simulink model "BLDCctrlBasedOnMBDPILmodel"  (R2020b)
settings: Solver=FixedStepDiscrete  StartTime=0.0  StopTime=10.0  FixedStep=0.0001  RelTol=1e-3
InitFcn:
  | mbd_s32k_consistency_checks(bdroot(gcs));
undefined symbols (not defined in the file or in its folder): LQFP
libraries: mbd_s32k1xx_ec_toolbox x16
settings Model: Creator=k  LastModifiedBy=k
settings DataIOCC: ExternalInput=off  InitialState=off  SaveOutput=off  SignalLogging=off  SaveTime=off
settings OptimizationCC: DefaultParameterBehavior=Inlined  EnhancedBackFolding=on  PassReuseOutputArgsAs=Individual arguments  ZeroExternalMemoryAtStartup=off  ZeroInternalMemoryAtStartup=off  OptimizeBlockOrder=speed  DifferentSizesBufferReuse=on  OptimizationCustomize=off  EfficientTunableParamExpr=on
settings DebuggingCC: InheritedTsInSrcMsg=none  SingleTaskRateTransMsg=error  ParameterTunabilityLossMsg=error  UnconnectedInputMsg=error  UnconnectedOutputMsg=error  UnconnectedLineMsg=error  UnknownTsInhSupMsg=error
settings HardwareCC: ProdBitPerPointer=32  ProdBitPerSizeT=32  ProdBitPerPtrDiffT=32  ProdLargestAtomicInteger=Long  ProdLargestAtomicFloat=Double  ProdWordSize=32  ProdHWDeviceType=ARM Compatible->ARM Cortex
settings SFSimCC: MATLABDynamicMemAlloc=off
settings RTWCC: Description=Model Based Design Toolbox S32K1xx Code Generation Target  SystemTargetFile=mbd_s32k.tlc  MakeCommand=mbd_s32k_make_rtw COPY_MDLREF_INCLUDES=0  TemplateMakefile=mbd_s32k.tmf
settings CodeAppCC: ForceParamTrailComments=on  IgnoreCustomStorageClasses=off  OperatorAnnotations=on  SimulinkDataObjDesc=on  SFDataObjDesc=on  InsertBlockDesc=on
settings STFCustomTargetCC: TargetLangStandard=C99 (ISO)  MultiwordLength=256  ConcurrentExecutionCompliant=off  CombineOutputUpdateFcns=on  ERTCustomFileBanners=on  SupportContinuousTime=off  SupportNonInlinedSFcns=off  RemoveResetFunc=on  MATLABClassNameForMDSCustomization=Simulink.SoftwareTarget.ERTCustomization  CPPClassGenCompliant=off  GRTInterface=off  SystemTargetFile=mbd_s32k.tlc
settings ERTTargetCC: TargetLangStandard=C99 (ISO)  ParMdlRefBuildCompliant=off  CompOptLevelCompliant=off  ConcurrentExecutionCompliant=off  ModelStepFunctionPrototypeControlCompliant=off  CPPClassGenCompliant=off  UseToolchainInfoCompliant=off  InlinedParameterPlacement=NonHierarchical  ERTSrcFileBannerTemplate=mbd_ert_code_template.cgt  ERTHdrFileBannerTemplate=mbd_ert_code_template.cgt  ERTDataSrcFileTemplate=mbd_ert_code_template.cgt  ERTDataHdrFileTemplate=mbd_ert_code_template.cgt  ERTCustomFileTemplate=example_file_process.tlc

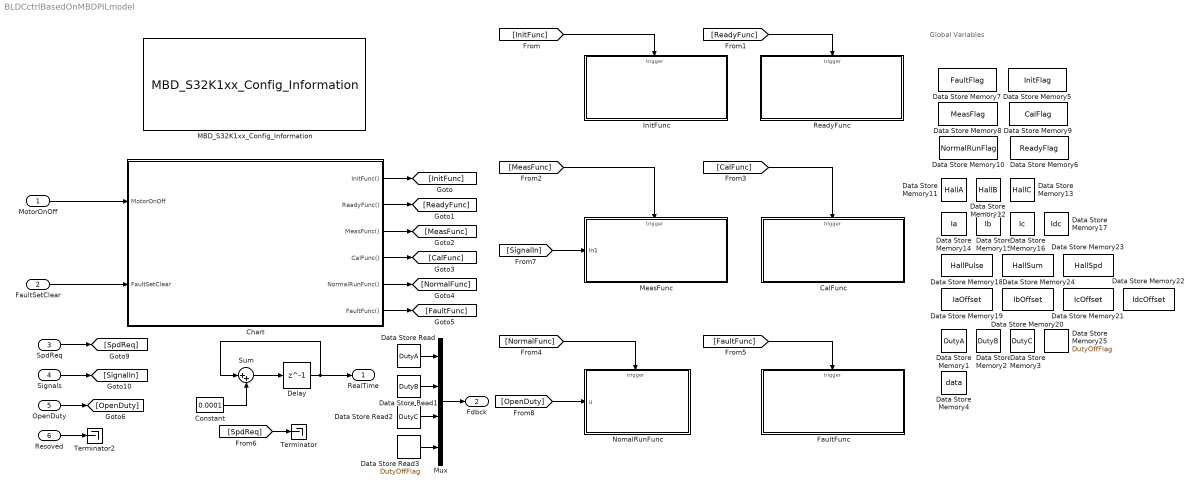
== system BLDCctrlBasedOnMBDPILmodel ==
  note: Global Variables
  MotorOnOff : Inport  OutDataTypeStr=boolean
  FaultSetClear : Inport  Port=2  OutDataTypeStr=boolean
  SpdReq : Inport  Port=3  OutDataTypeStr=single
  Signals : Inport  Port=4  OutDataTypeStr=single  PortDimensions=7
  OpenDuty : Inport  Port=5  OutDataTypeStr=single
  Resoved : Inport  Port=6  OutDataTypeStr=single
  CalFunc : Subsystem  TreatAsAtomicUnit=on
  Chart : Stateflow chart  TreatAsAtomicUnit=on
      settings: PortSchema="{\"entries\":[{\"content\":{\"sides\":[{\"content\":{\"connectorIds\":[\"In1\",\"In2\"]},\"type\":\"ConnectorPlacement.EquallySpacedRectSide\",\"uuid\":\"6aab3670-dbd5-4778-9051-de706f320d6c\"},{\"content\":{\"connectorIds\":[\"Out2\",\"Out3\",\"Out1\",\"Out4\",\"Out5\",\"Out6\"],\"side\":\"RIGHT\"},\"type\":\"ConnectorPlacement.EquallySpacedRectSide\",\"uuid\":\"2f9f0170-7a01-4f36-b182-da63b20b6c86\"},{\"content\":{\"connectorIds\":[],\"side\":\"TOP\"},\"type\":\"ConnectorPlacement.EquallySpacedRectSide\",\"uuid\":\"ed2088fa-8282-455e-b501-bc381afe58e4\"},{\"content\":{\"connectorIds\":[],\"side\":\"HIDDEN\"},\"type\":\"ConnectorPlacement.EquallySpacedRectSide\",\"uuid\":\"d652818b-6052-4db5-9e3c-1b8d8b3f5bf8\"}]},\"type\":\"ConnectorPlacement.EquallySpacedConnector\",\"uuid\":\"e57e4f41-1290-4580-a9fc-0c62073a8c32\"}],\"packageUris\":[\"http://schema.mathworks.com/mf0/Connector/R2020b\"],\"version\":\"1.0\"}"
  Constant : Constant  Value=0.0001  OutDataTypeStr=single
  Data Store Memory1 : DataStoreMemory  DataStoreName=DutyA  ReadBeforeWriteMsg=warning  WriteAfterWriteMsg=warning  WriteAfterReadMsg=warning  ShowAdditionalParam=off
  Data Store Memory10 : DataStoreMemory  DataStoreName=NormalRunFlag  ReadBeforeWriteMsg=warning  WriteAfterWriteMsg=warning  WriteAfterReadMsg=warning  ShowAdditionalParam=off
  Data Store Memory11 : DataStoreMemory  DataStoreName=HallA  ReadBeforeWriteMsg=warning  WriteAfterWriteMsg=warning  WriteAfterReadMsg=warning  ShowAdditionalParam=off  OutDataTypeStr=boolean
  Data Store Memory12 : DataStoreMemory  DataStoreName=HallB  ReadBeforeWriteMsg=warning  WriteAfterWriteMsg=warning  WriteAfterReadMsg=warning  ShowAdditionalParam=off  OutDataTypeStr=boolean
  Data Store Memory13 : DataStoreMemory  DataStoreName=HallC  ReadBeforeWriteMsg=warning  WriteAfterWriteMsg=warning  WriteAfterReadMsg=warning  ShowAdditionalParam=off  OutDataTypeStr=boolean
  Data Store Memory14 : DataStoreMemory  DataStoreName=Ia  ReadBeforeWriteMsg=warning  WriteAfterWriteMsg=warning  WriteAfterReadMsg=warning  ShowAdditionalParam=off
  Data Store Memory15 : DataStoreMemory  DataStoreName=Ib  ReadBeforeWriteMsg=warning  WriteAfterWriteMsg=warning  WriteAfterReadMsg=warning  ShowAdditionalParam=off
  Data Store Memory16 : DataStoreMemory  DataStoreName=Ic  ReadBeforeWriteMsg=warning  WriteAfterWriteMsg=warning  WriteAfterReadMsg=warning  ShowAdditionalParam=off
  Data Store Memory17 : DataStoreMemory  DataStoreName=Idc  ReadBeforeWriteMsg=warning  WriteAfterWriteMsg=warning  WriteAfterReadMsg=warning  ShowAdditionalParam=off
  Data Store Memory18 : DataStoreMemory  DataStoreName=HallPulse  ReadBeforeWriteMsg=warning  WriteAfterWriteMsg=warning  WriteAfterReadMsg=warning  ShowAdditionalParam=off  OutDataTypeStr=boolean
  Data Store Memory19 : DataStoreMemory  DataStoreName=IaOffset  ReadBeforeWriteMsg=warning  WriteAfterWriteMsg=warning  WriteAfterReadMsg=warning  ShowAdditionalParam=off
  Data Store Memory2 : DataStoreMemory  DataStoreName=DutyB  ReadBeforeWriteMsg=warning  WriteAfterWriteMsg=warning  WriteAfterReadMsg=warning  ShowAdditionalParam=off
  Data Store Memory20 : DataStoreMemory  DataStoreName=IbOffset  ReadBeforeWriteMsg=warning  WriteAfterWriteMsg=warning  WriteAfterReadMsg=warning  ShowAdditionalParam=off
  Data Store Memory21 : DataStoreMemory  DataStoreName=IcOffset  ReadBeforeWriteMsg=warning  WriteAfterWriteMsg=warning  WriteAfterReadMsg=warning  ShowAdditionalParam=off
  Data Store Memory22 : DataStoreMemory  DataStoreName=IdcOffset  ReadBeforeWriteMsg=warning  WriteAfterWriteMsg=warning  WriteAfterReadMsg=warning  ShowAdditionalParam=off
  Data Store Memory23 : DataStoreMemory  DataStoreName=HallSpd  ReadBeforeWriteMsg=warning  WriteAfterWriteMsg=warning  WriteAfterReadMsg=warning  ShowAdditionalParam=off
  Data Store Memory24 : DataStoreMemory  DataStoreName=HallSum  ReadBeforeWriteMsg=warning  WriteAfterWriteMsg=warning  WriteAfterReadMsg=warning  ShowAdditionalParam=off  OutDataTypeStr=single
  Data Store Memory25 : DataStoreMemory  DataStoreName=DutyOffFlag  ReadBeforeWriteMsg=warning  WriteAfterWriteMsg=warning  WriteAfterReadMsg=warning  ShowAdditionalParam=off
  Data Store Memory3 : DataStoreMemory  DataStoreName=DutyC  ReadBeforeWriteMsg=warning  WriteAfterWriteMsg=warning  WriteAfterReadMsg=warning  ShowAdditionalParam=off
  Data Store Memory4 : DataStoreMemory  DataStoreName=data  ReadBeforeWriteMsg=warning  WriteAfterWriteMsg=warning  WriteAfterReadMsg=warning  ShowAdditionalParam=off
  Data Store Memory5 : DataStoreMemory  DataStoreName=InitFlag  ReadBeforeWriteMsg=warning  WriteAfterWriteMsg=warning  WriteAfterReadMsg=warning  ShowAdditionalParam=off
  Data Store Memory6 : DataStoreMemory  DataStoreName=ReadyFlag  ReadBeforeWriteMsg=warning  WriteAfterWriteMsg=warning  WriteAfterReadMsg=warning  ShowAdditionalParam=off
  Data Store Memory7 : DataStoreMemory  DataStoreName=FaultFlag  ReadBeforeWriteMsg=warning  WriteAfterWriteMsg=warning  WriteAfterReadMsg=warning  ShowAdditionalParam=off
  Data Store Memory8 : DataStoreMemory  DataStoreName=MeasFlag  ReadBeforeWriteMsg=warning  WriteAfterWriteMsg=warning  WriteAfterReadMsg=warning  ShowAdditionalParam=off
  Data Store Memory9 : DataStoreMemory  DataStoreName=CalFlag  ReadBeforeWriteMsg=warning  WriteAfterWriteMsg=warning  WriteAfterReadMsg=warning  ShowAdditionalParam=off
  Data Store Read : DataStoreRead  DataStoreName=DutyA
  Data Store Read1 : DataStoreRead  DataStoreName=DutyB
  Data Store Read2 : DataStoreRead  DataStoreName=DutyC
  Data Store Read3 : DataStoreRead  DataStoreName=DutyOffFlag
  Delay : Delay  DelayLength=1  InitialCondition=0
  FaultFunc : Subsystem  TreatAsAtomicUnit=on
  InitFunc : Subsystem  TreatAsAtomicUnit=on
  MBD_S32K1xx_Config_Information : mbd_s32k1xx_ec_toolbox/MBD_S32K1xx_Config_Information  mbdt_ver=0  disp_str=|  config_params=[]  mcu_target_name=S32K144  mcu_target_package=100-LQFP  mcu_target_sram_size=64KB  mcu_system_clock_freq=80  mcu_xtal_freq=External 8  mcu_steptick_timer=LPIT Channel 0  mcu_steptick_prio=15  ds_import_enable=on  target_compiler=GCC  target_memory=FLASH  gcc_target_compile_opts=-mthumb -mfloat-abi=hard -mfpu=fpv4-sp-d16 -O1 -g -gstrict-dwarf  gcc_target_assemble_opts=-mthumb -mfloat-abi=hard -mfpu=fpv4-sp-d16 -g  gcc_target_link_opts=-mthumb -mfloat-abi=hard -mfpu=fpv4-sp-d16  gcc_target_default_lcf=on  gcc_target_user_lcf=S32K148_192_flash.ld  ghs_target_compile_opts=-cpu=cortexm4f -thumb -fpu=vfpv4_d16 -fsingle -Ogeneral -Wundef -Wimplicit-int -Wshadow -Wtrigraphs --no_commons --gnu_asm -gnu99 -gdwarf-2 -G  ghs_target_assemble_opts=-cpu=cortexm4f -fpu=vfpv4_d16  ghs_target_link_opts=-cpu=cortexm4f -thumb -fpu=vfpv4_d16  ghs_target_default_lcf=on  ghs_target_user_lcf=S32K148_192_flash.ld  iar_target_compile_opts=--cpu=Cortex-M4F --thumb --fpu=VFPv4_sp -Ol -e --debug --dlib_config normal  iar_target_assemble_opts=--cpu Cortex-M4F --thumb --fpu VFPv4_sp  iar_target_link_opts=--no_exceptions --vfe --inline  iar_target_default_lcf=on  iar_target_user_lcf=S32K148_192_flash.icf  pil_download_enable=on  rbl_download_enable=off  rbl_start_delay=5000  rbl_download_interface=OpenSDA  rbl_restart_request=off  rbl_com_port=COM6  rbl_com_port_custom=COM1  pil_download_rate=57600  pil_opensda_drive=Custom  pil_opensda_drive_custom=E  pil_uart_instance=1  pil_uart_rx=PTC6: [LPUART1_RX | Receive]  pil_uart_tx=PTC7: [LPUART1_TX | Transmit]  FTM_PWM_PcrCheckEnDis=on  FTM_Input_Edge_Inputs_PcrCheckEnDis=on  FTM_Dual_Edge_Inputs_PcrCheckEnDis=on  FTM_Quadrature_Inputs_PcrCheckEnDis=on  FTM_Hall_Sensor_Inputs_PcrCheckEnDis=on  LPTMR_PcrCheckEnDis=on  PIT_PcrCheckEnDis=on  RTC_PcrCheckEnDis=on  FlexCAN_PcrCheckEnDis=on  LIN_PcrCheckEnDis=on  FlexIO_PcrCheckEnDis=on  LPI2C_PcrCheckEnDis=on  LPSPI_PcrCheckEnDis=on  LPUART_PcrCheckEnDis=on  CMP_PcrCheckEnDis=on  GPIO_OutputPcrCheckEnDis=on  GPIO_InputPcrCheckEnDis=on  SBC_PcrCheckEnDis=on  BMS_PcrCheckEnDis=on  AMMCLIB_PcrCheckEnDis=on  FM_PcrCheckEnDis=on  Profile_PcrCheckEnDis=on  ConfigParams_PcrCheckEnDis=on  ModelRef_PcrCheckEnDis=on  PDB0_PcrCheckEnDis=on  CSEc_PcrCheckEnDis=on  eDMA_PcrCheckEnDis=on  FLASH_PcrCheckEnDis=on  ADC_PcrCheckEnDis=on  WDOG_PcrCheckEnDis=on
      | Target : S32K144-64KB_SRAM
      | Package : 100-pin
      | System clock : 80 MHz
      | XTAL clock : External 8 MHz
      | Compiler : IAR
      | Target Type : FLASH
      | Download Code after build : off
      | Step Tick Interrupt Priority : 15
  MeasFunc : Subsystem  TreatAsAtomicUnit=on
  Mux : Mux
  NomalRunFunc : Subsystem  TreatAsAtomicUnit=on
  ReadyFunc : Subsystem  TreatAsAtomicUnit=on
  Sum : Sum  Inputs=|++
  Terminator : Terminator
  Terminator2 : Terminator
  RealTime : Outport  OutDataTypeStr=single
  Fdbck : Outport  Port=2  OutDataTypeStr=single  PortDimensions=4
  wires:
  MotorOnOff/1 -> Chart/1(MotorOnOff)
  FaultSetClear/1 -> Chart/2(FaultSetClear)
  SpdReq/1 -> [SpdReq]
  Signals/1 -> [SignalIn]
  OpenDuty/1 -> [OpenDuty]
  Resoved/1 -> Terminator2/1
  Chart/2(InitFunc()) -> [InitFunc]
  Chart/3(ReadyFunc()) -> [ReadyFunc]
  Chart/1(MeasFunc()) -> [MeasFunc]
  Chart/4(CalFunc()) -> [CalFunc]
  Chart/6(FaultFunc()) -> [FaultFunc]
  Chart/5(NormalRunFunc()) -> [NormalFunc]
  [ReadyFunc] -> ReadyFunc/Trigger
  [InitFunc] -> InitFunc/Trigger
  [MeasFunc] -> MeasFunc/Trigger
  [FaultFunc] -> FaultFunc/Trigger
  [CalFunc] -> CalFunc/Trigger
  [NormalFunc] -> NomalRunFunc/Trigger
  [SignalIn] -> MeasFunc/1(In1)
  Sum/1 -> Delay/1
  Constant/1 -> Sum/2
  Delay/1 -> Sum/1, RealTime/1
  [OpenDuty] -> NomalRunFunc/1(u)
  Data Store Read/1 -> Mux/1
  Data Store Read1/1 -> Mux/2
  Data Store Read2/1 -> Mux/3
  Data Store Read3/1 -> Mux/4
  Mux/1 -> Fdbck/1
  [SpdReq] -> Terminator/1

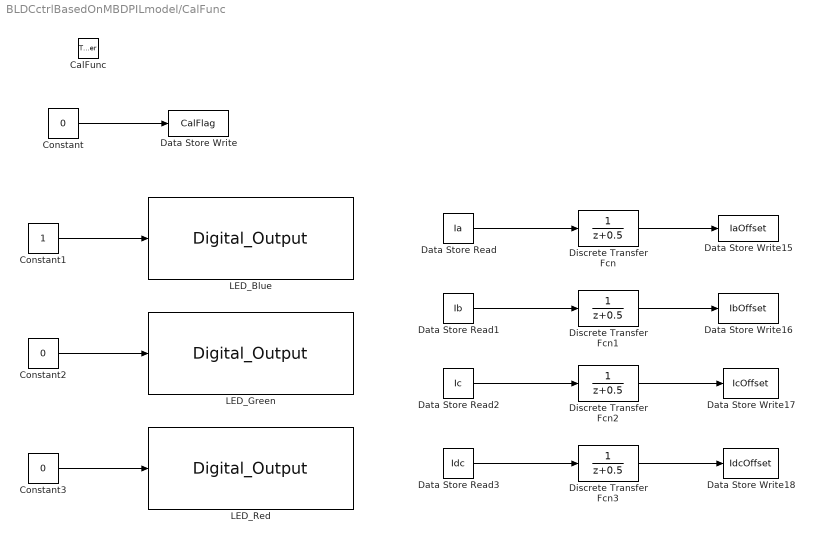
== system BLDCctrlBasedOnMBDPILmodel/CalFunc ==
  CalFunc : TriggerPort  TriggerType=function-call  VariantControl=Variant
  Constant : Constant  Value=0  OutDataTypeStr=boolean
  Constant1 : Constant  OutDataTypeStr=boolean
  Constant2 : Constant  Value=0  OutDataTypeStr=boolean
  Constant3 : Constant  Value=0  OutDataTypeStr=boolean
  Data Store Read : DataStoreRead  DataStoreName=Ia
  Data Store Read1 : DataStoreRead  DataStoreName=Ib
  Data Store Read2 : DataStoreRead  DataStoreName=Ic
  Data Store Read3 : DataStoreRead  DataStoreName=Idc
  Data Store Write : DataStoreWrite  DataStoreName=CalFlag
  Data Store Write15 : DataStoreWrite  DataStoreName=IaOffset
  Data Store Write16 : DataStoreWrite  DataStoreName=IbOffset
  Data Store Write17 : DataStoreWrite  DataStoreName=IcOffset
  Data Store Write18 : DataStoreWrite  DataStoreName=IdcOffset
  Discrete Transfer Fcn{,1..3} (4 alike) : DiscreteTransferFcn
  LED_Blue : mbd_s32k1xx_ec_toolbox/GPIO Blocks/Digital_Output  gpio_pin=PTD0: [PTD0 | Port D I/O]  init_val=Low  drive_strength=Low
  LED_Green : mbd_s32k1xx_ec_toolbox/GPIO Blocks/Digital_Output  gpio_pin=PTD16: [PTD16 | Port D I/O]  init_val=Low  drive_strength=Low
  LED_Red : mbd_s32k1xx_ec_toolbox/GPIO Blocks/Digital_Output  gpio_pin=PTD15: [PTD15 | Port D I/O]  init_val=Low  drive_strength=Low
  wires:
  Constant/1 -> Data Store Write/1
  Constant2/1 -> LED_Green/1
  Constant3/1 -> LED_Red/1
  Constant1/1 -> LED_Blue/1
  Data Store Read/1 -> Discrete Transfer Fcn/1
  Data Store Read1/1 -> Discrete Transfer Fcn1/1
  Data Store Read2/1 -> Discrete Transfer Fcn2/1
  Data Store Read3/1 -> Discrete Transfer Fcn3/1
  Discrete Transfer Fcn/1 -> Data Store Write15/1
  Discrete Transfer Fcn1/1 -> Data Store Write16/1
  Discrete Transfer Fcn2/1 -> Data Store Write17/1
  Discrete Transfer Fcn3/1 -> Data Store Write18/1

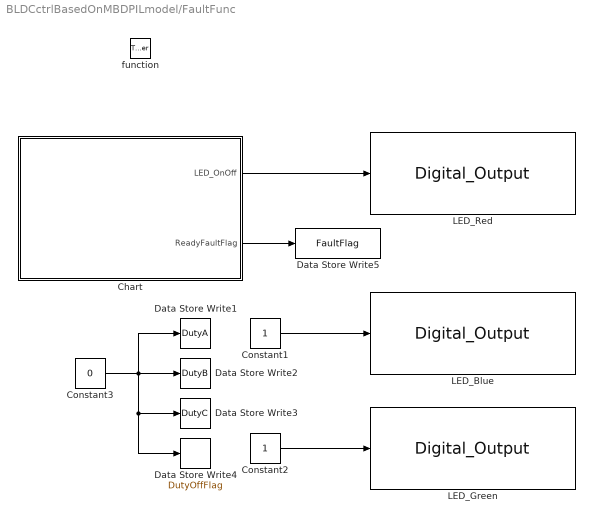
== system BLDCctrlBasedOnMBDPILmodel/FaultFunc ==
  function : TriggerPort  TriggerType=function-call  VariantControl=Variant
  Chart : Stateflow chart  TreatAsAtomicUnit=on
  Constant1 : Constant  OutDataTypeStr=boolean
  Constant2 : Constant  OutDataTypeStr=boolean
  Constant3 : Constant  Value=0  OutDataTypeStr=single
  Data Store Write1 : DataStoreWrite  DataStoreName=DutyA
  Data Store Write2 : DataStoreWrite  DataStoreName=DutyB
  Data Store Write3 : DataStoreWrite  DataStoreName=DutyC
  Data Store Write4 : DataStoreWrite  DataStoreName=DutyOffFlag
  Data Store Write5 : DataStoreWrite  DataStoreName=FaultFlag
  LED_Blue : mbd_s32k1xx_ec_toolbox/GPIO Blocks/Digital_Output  gpio_pin=PTD0: [PTD0 | Port D I/O]  init_val=Low  drive_strength=Low
  LED_Green : mbd_s32k1xx_ec_toolbox/GPIO Blocks/Digital_Output  gpio_pin=PTD16: [PTD16 | Port D I/O]  init_val=Low  drive_strength=Low
  LED_Red : mbd_s32k1xx_ec_toolbox/GPIO Blocks/Digital_Output  gpio_pin=PTD15: [PTD15 | Port D I/O]  init_val=Low  drive_strength=Low
  wires:
  Chart/2(ReadyFaultFlag) -> Data Store Write5/1
  Chart/1(LED_OnOff) -> LED_Red/1
  Constant2/1 -> LED_Green/1
  Constant1/1 -> LED_Blue/1
  Constant3/1 -> Data Store Write1/1, Data Store Write2/1, Data Store Write4/1, Data Store Write3/1

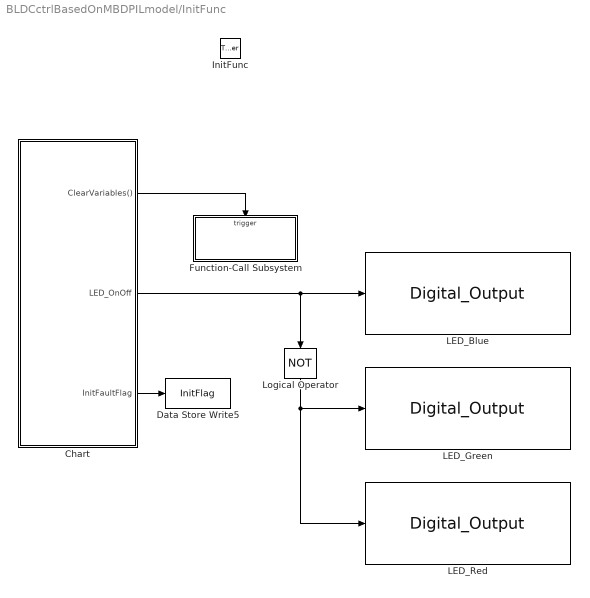
== system BLDCctrlBasedOnMBDPILmodel/InitFunc ==
  InitFunc : TriggerPort  TriggerType=function-call  VariantControl=Variant
  Chart : Stateflow chart  TreatAsAtomicUnit=on
      settings: PortSchema="{\"entries\":[{\"content\":{\"sides\":[{\"content\":{\"connectorIds\":[]},\"type\":\"ConnectorPlacement.EquallySpacedRectSide\",\"uuid\":\"354d3f51-1e42-4f8f-b10a-6144ae9b16f3\"},{\"content\":{\"connectorIds\":[\"Out3\",\"Out1\",\"Out2\"],\"side\":\"RIGHT\"},\"type\":\"ConnectorPlacement.EquallySpacedRectSide\",\"uuid\":\"2d24ccff-5c9c-4bc9-a1dd-d33dfcc71136\"},{\"content\":{\"connectorIds\":[],\"side\":\"TOP\"},\"type\":\"ConnectorPlacement.EquallySpacedRectSide\",\"uuid\":\"341841bf-8a4d-414a-80d5-e0f59e48ceb5\"},{\"content\":{\"connectorIds\":[],\"side\":\"HIDDEN\"},\"type\":\"ConnectorPlacement.EquallySpacedRectSide\",\"uuid\":\"f114981b-6163-49e2-8927-8024c343f032\"}]},\"type\":\"ConnectorPlacement.EquallySpacedConnector\",\"uuid\":\"cb0f31e5-98f2-4141-900a-6a24dbca6936\"}],\"packageUris\":[\"http://schema.mathworks.com/mf0/Connector/R2020b\"],\"version\":\"1.0\"}"
  Data Store Write5 : DataStoreWrite  DataStoreName=InitFlag
  Function-Call Subsystem : Subsystem  TreatAsAtomicUnit=on
  LED_Blue : mbd_s32k1xx_ec_toolbox/GPIO Blocks/Digital_Output  gpio_pin=PTD0: [PTD0 | Port D I/O]  init_val=Low  drive_strength=Low
  LED_Green : mbd_s32k1xx_ec_toolbox/GPIO Blocks/Digital_Output  gpio_pin=PTD16: [PTD16 | Port D I/O]  init_val=Low  drive_strength=Low
  LED_Red : mbd_s32k1xx_ec_toolbox/GPIO Blocks/Digital_Output  gpio_pin=PTD15: [PTD15 | Port D I/O]  init_val=Low  drive_strength=Low
  Logical Operator : Logic  Operator=NOT  AllPortsSameDT=off  OutDataTypeStr=boolean
  wires:
  Chart/1(LED_OnOff) -> LED_Blue/1, Logical Operator/1
  Chart/2(InitFaultFlag) -> Data Store Write5/1
  Logical Operator/1 -> LED_Red/1, LED_Green/1
  Chart/3(ClearVariables()) -> Function-Call Subsystem/Trigger

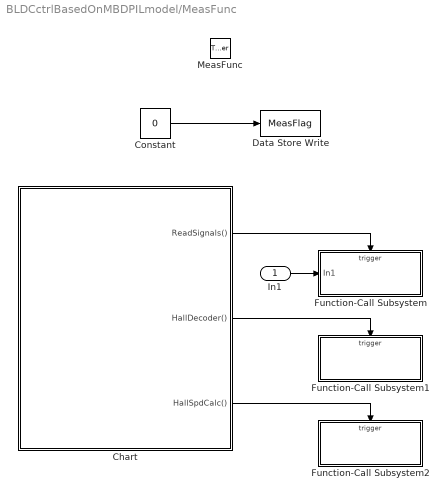
== system BLDCctrlBasedOnMBDPILmodel/MeasFunc ==
  In1 : Inport
  MeasFunc : TriggerPort  TriggerType=function-call  VariantControl=Variant
  Chart : Stateflow chart  TreatAsAtomicUnit=on
  Constant : Constant  Value=0  OutDataTypeStr=boolean
  Data Store Write : DataStoreWrite  DataStoreName=MeasFlag
  Function-Call Subsystem : Subsystem  TreatAsAtomicUnit=on
  Function-Call Subsystem1 : Subsystem  TreatAsAtomicUnit=on
  Function-Call Subsystem2 : Subsystem  TreatAsAtomicUnit=on
  wires:
  Constant/1 -> Data Store Write/1
  Chart/1(ReadSignals()) -> Function-Call Subsystem/Trigger
  In1/1 -> Function-Call Subsystem/1(In1)
  Chart/2(HallDecoder()) -> Function-Call Subsystem1/Trigger
  Chart/3(HallSpdCalc()) -> Function-Call Subsystem2/Trigger

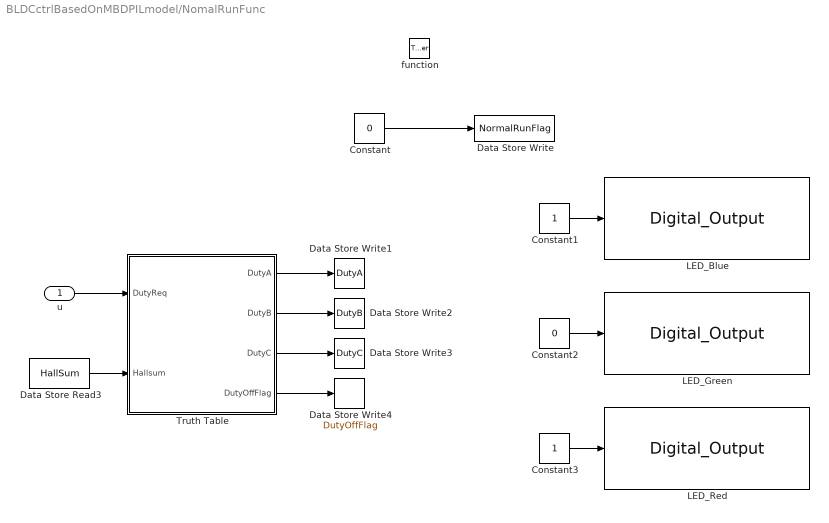
== system BLDCctrlBasedOnMBDPILmodel/NomalRunFunc ==
  u : Inport
  function : TriggerPort  TriggerType=function-call  VariantControl=Variant
  Constant : Constant  Value=0  OutDataTypeStr=boolean
  Constant1 : Constant  OutDataTypeStr=boolean
  Constant2 : Constant  Value=0  OutDataTypeStr=boolean
  Constant3 : Constant  OutDataTypeStr=boolean
  Data Store Read3 : DataStoreRead  DataStoreName=HallSum
  Data Store Write : DataStoreWrite  DataStoreName=NormalRunFlag
  Data Store Write1 : DataStoreWrite  DataStoreName=DutyA
  Data Store Write2 : DataStoreWrite  DataStoreName=DutyB
  Data Store Write3 : DataStoreWrite  DataStoreName=DutyC
  Data Store Write4 : DataStoreWrite  DataStoreName=DutyOffFlag
  LED_Blue : mbd_s32k1xx_ec_toolbox/GPIO Blocks/Digital_Output  gpio_pin=PTD0: [PTD0 | Port D I/O]  init_val=Low  drive_strength=Low
  LED_Green : mbd_s32k1xx_ec_toolbox/GPIO Blocks/Digital_Output  gpio_pin=PTD16: [PTD16 | Port D I/O]  init_val=Low  drive_strength=Low
  LED_Red : mbd_s32k1xx_ec_toolbox/GPIO Blocks/Digital_Output  gpio_pin=PTD15: [PTD15 | Port D I/O]  init_val=Low  drive_strength=Low
  Truth Table : Truth Table  TreatAsAtomicUnit=on
      settings: PortSchema="{\"entries\":[{\"content\":{\"sides\":[{\"content\":{\"connectorIds\":[\"In2\",\"In1\"]},\"type\":\"ConnectorPlacement.EquallySpacedRectSide\",\"uuid\":\"59c0d94d-4ab6-4082-9c20-9efdae7878b3\"},{\"content\":{\"connectorIds\":[\"Out1\",\"Out2\",\"Out3\",\"Out4\"],\"side\":\"RIGHT\"},\"type\":\"ConnectorPlacement.EquallySpacedRectSide\",\"uuid\":\"fbebaf7f-5920-4df9-84a7-9b0467c91c72\"},{\"content\":{\"connectorIds\":[],\"side\":\"TOP\"},\"type\":\"ConnectorPlacement.EquallySpacedRectSide\",\"uuid\":\"8ff1c87b-d4dc-46a0-9459-25a6278b9f20\"},{\"content\":{\"connectorIds\":[],\"side\":\"HIDDEN\"},\"type\":\"ConnectorPlacement.EquallySpacedRectSide\",\"uuid\":\"16bdd2e1-f1a8-43ed-aa1c-d33053eb9e05\"}]},\"type\":\"ConnectorPlacement.EquallySpacedConnector\",\"uuid\":\"7896656f-e18e-44d5-80e3-9050e65d4579\"}],\"packageUris\":[\"http://schema.mathworks.com/mf0/Connector/R2020b\"],\"version\":\"1.0\"}"
  wires:
  Constant/1 -> Data Store Write/1
  Constant1/1 -> LED_Blue/1
  Constant2/1 -> LED_Green/1
  Constant3/1 -> LED_Red/1
  Data Store Read3/1 -> Truth Table/1(Hallsum)
  Truth Table/1(DutyA) -> Data Store Write1/1
  Truth Table/3(DutyC) -> Data Store Write3/1
  u/1 -> Truth Table/2(DutyReq)
  Truth Table/2(DutyB) -> Data Store Write2/1
  Truth Table/4(DutyOffFlag) -> Data Store Write4/1

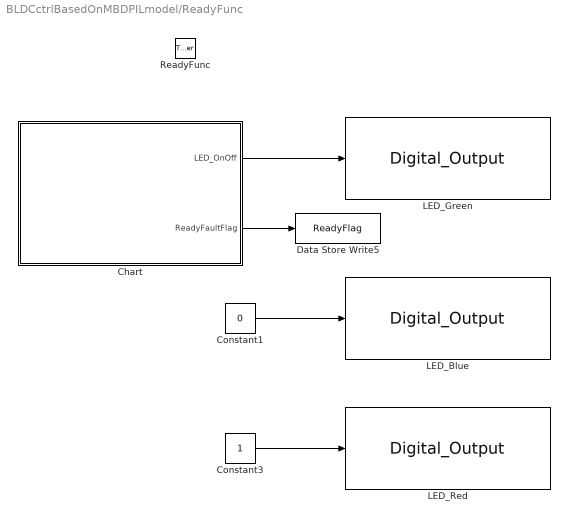
== system BLDCctrlBasedOnMBDPILmodel/ReadyFunc ==
  ReadyFunc : TriggerPort  TriggerType=function-call  VariantControl=Variant
  Chart : Stateflow chart  TreatAsAtomicUnit=on
  Constant1 : Constant  Value=0  OutDataTypeStr=boolean
  Constant3 : Constant  OutDataTypeStr=boolean
  Data Store Write5 : DataStoreWrite  DataStoreName=ReadyFlag
  LED_Blue : mbd_s32k1xx_ec_toolbox/GPIO Blocks/Digital_Output  gpio_pin=PTD0: [PTD0 | Port D I/O]  init_val=Low  drive_strength=Low
  LED_Green : mbd_s32k1xx_ec_toolbox/GPIO Blocks/Digital_Output  gpio_pin=PTD16: [PTD16 | Port D I/O]  init_val=Low  drive_strength=Low
  LED_Red : mbd_s32k1xx_ec_toolbox/GPIO Blocks/Digital_Output  gpio_pin=PTD15: [PTD15 | Port D I/O]  init_val=Low  drive_strength=Low
  wires:
  Chart/2(ReadyFaultFlag) -> Data Store Write5/1
  Chart/1(LED_OnOff) -> LED_Green/1
  Constant3/1 -> LED_Red/1
  Constant1/1 -> LED_Blue/1

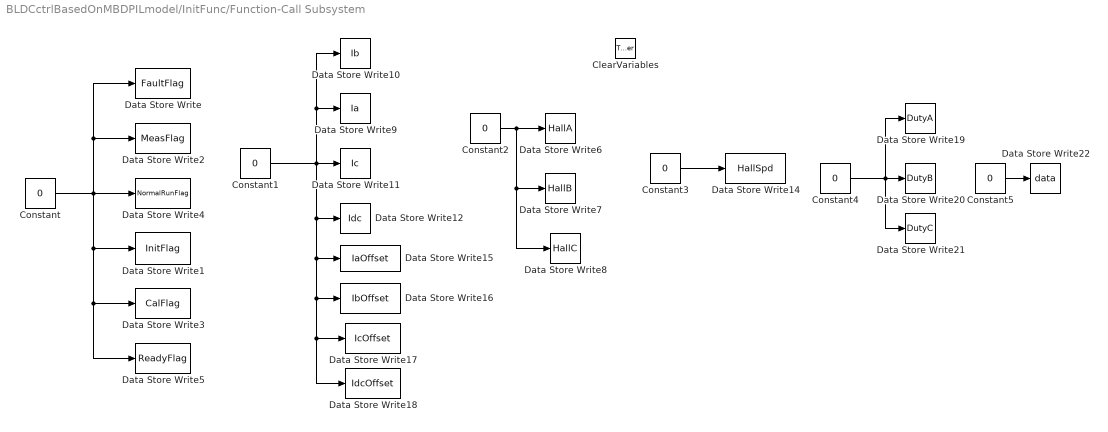
== system BLDCctrlBasedOnMBDPILmodel/InitFunc/Function-Call Subsystem ==
  ClearVariables : TriggerPort  TriggerType=function-call  VariantControl=Variant
  Constant : Constant  Value=0  OutDataTypeStr=boolean
  Constant{1,3..5} (4 alike) : Constant  Value=0  OutDataTypeStr=single
  Constant2 : Constant  Value=0  OutDataTypeStr=boolean
  Data Store Write : DataStoreWrite  DataStoreName=FaultFlag
  Data Store Write1 : DataStoreWrite  DataStoreName=InitFlag
  Data Store Write10 : DataStoreWrite  DataStoreName=Ib
  Data Store Write11 : DataStoreWrite  DataStoreName=Ic
  Data Store Write12 : DataStoreWrite  DataStoreName=Idc
  Data Store Write14 : DataStoreWrite  DataStoreName=HallSpd
  Data Store Write15 : DataStoreWrite  DataStoreName=IaOffset
  Data Store Write16 : DataStoreWrite  DataStoreName=IbOffset
  Data Store Write17 : DataStoreWrite  DataStoreName=IcOffset
  Data Store Write18 : DataStoreWrite  DataStoreName=IdcOffset
  Data Store Write19 : DataStoreWrite  DataStoreName=DutyA
  Data Store Write2 : DataStoreWrite  DataStoreName=MeasFlag
  Data Store Write20 : DataStoreWrite  DataStoreName=DutyB
  Data Store Write21 : DataStoreWrite  DataStoreName=DutyC
  Data Store Write22 : DataStoreWrite  DataStoreName=data
  Data Store Write3 : DataStoreWrite  DataStoreName=CalFlag
  Data Store Write4 : DataStoreWrite  DataStoreName=NormalRunFlag
  Data Store Write5 : DataStoreWrite  DataStoreName=ReadyFlag
  Data Store Write6 : DataStoreWrite  DataStoreName=HallA
  Data Store Write7 : DataStoreWrite  DataStoreName=HallB
  Data Store Write8 : DataStoreWrite  DataStoreName=HallC
  Data Store Write9 : DataStoreWrite  DataStoreName=Ia
  wires:
  Constant/1 -> Data Store Write/1, Data Store Write2/1, Data Store Write5/1, Data Store Write3/1, Data Store Write1/1, Data Store Write4/1
  Constant1/1 -> Data Store Write10/1, Data Store Write9/1, Data Store Write11/1, Data Store Write12/1, Data Store Write15/1, Data Store Write16/1, Data Store Write17/1, Data Store Write18/1
  Constant2/1 -> Data Store Write8/1, Data Store Write7/1, Data Store Write6/1
  Constant3/1 -> Data Store Write14/1
  Constant4/1 -> Data Store Write19/1, Data Store Write21/1, Data Store Write20/1
  Constant5/1 -> Data Store Write22/1

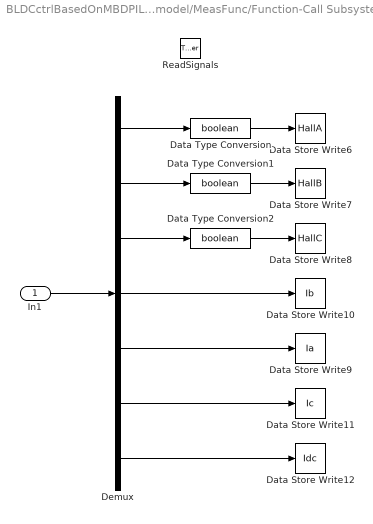
== system BLDCctrlBasedOnMBDPILmodel/MeasFunc/Function-Call Subsystem ==
  In1 : Inport
  ReadSignals : TriggerPort  TriggerType=function-call  VariantControl=Variant
  Data Store Write10 : DataStoreWrite  DataStoreName=Ib
  Data Store Write11 : DataStoreWrite  DataStoreName=Ic
  Data Store Write12 : DataStoreWrite  DataStoreName=Idc
  Data Store Write6 : DataStoreWrite  DataStoreName=HallA
  Data Store Write7 : DataStoreWrite  DataStoreName=HallB
  Data Store Write8 : DataStoreWrite  DataStoreName=HallC
  Data Store Write9 : DataStoreWrite  DataStoreName=Ia
  Data Type Conversion : DataTypeConversion  OutDataTypeStr=boolean
  Data Type Conversion1 : DataTypeConversion  OutDataTypeStr=boolean
  Data Type Conversion2 : DataTypeConversion  OutDataTypeStr=boolean
  Demux : Demux  Outputs=7
  wires:
  Demux/5 -> Data Store Write9/1
  Demux/3 -> Data Type Conversion2/1
  Demux/2 -> Data Type Conversion1/1
  Demux/4 -> Data Store Write10/1
  In1/1 -> Demux/1
  Demux/7 -> Data Store Write12/1
  Demux/6 -> Data Store Write11/1
  Data Type Conversion1/1 -> Data Store Write7/1
  Data Type Conversion2/1 -> Data Store Write8/1
  Demux/1 -> Data Type Conversion/1
  Data Type Conversion/1 -> Data Store Write6/1

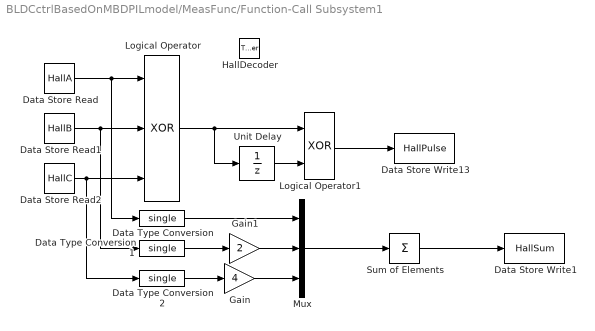
== system BLDCctrlBasedOnMBDPILmodel/MeasFunc/Function-Call Subsystem1 ==
  HallDecoder : TriggerPort  TriggerType=function-call  VariantControl=Variant
  Data Store Read : DataStoreRead  DataStoreName=HallA
  Data Store Read1 : DataStoreRead  DataStoreName=HallB
  Data Store Read2 : DataStoreRead  DataStoreName=HallC
  Data Store Write1 : DataStoreWrite  DataStoreName=HallSum
  Data Store Write13 : DataStoreWrite  DataStoreName=HallPulse
  Data Type Conversion : DataTypeConversion  OutDataTypeStr=single
  Data Type Conversion1 : DataTypeConversion  OutDataTypeStr=single
  Data Type Conversion2 : DataTypeConversion  OutDataTypeStr=single
  Gain : Gain  Gain=4
  Gain1 : Gain  Gain=2
  Logical Operator : Logic  Operator=XOR  Inputs=3  AllPortsSameDT=off  OutDataTypeStr=boolean
  Logical Operator1 : Logic  Operator=XOR  AllPortsSameDT=off  OutDataTypeStr=boolean
  Mux : Mux  Inputs=3
  Sum of Elements : Sum  Inputs=+
  Unit Delay : UnitDelay  SampleTime=-1  HasFrameUpgradeWarning=on
  wires:
  Data Store Read/1 -> Data Type Conversion/1, Logical Operator/1
  Data Store Read2/1 -> Data Type Conversion2/1, Logical Operator/3
  Logical Operator/1 -> Logical Operator1/1, Unit Delay/1
  Unit Delay/1 -> Logical Operator1/2
  Logical Operator1/1 -> Data Store Write13/1
  Gain/1 -> Mux/3
  Gain1/1 -> Mux/2
  Mux/1 -> Sum of Elements/1
  Sum of Elements/1 -> Data Store Write1/1
  Data Type Conversion/1 -> Mux/1
  Data Store Read1/1 -> Data Type Conversion1/1, Logical Operator/2
  Data Type Conversion1/1 -> Gain1/1
  Data Type Conversion2/1 -> Gain/1

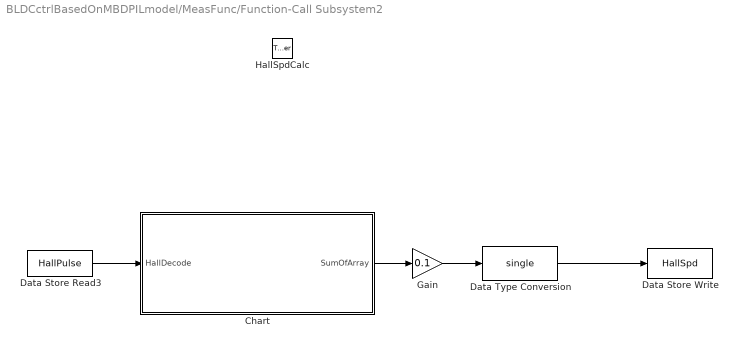
== system BLDCctrlBasedOnMBDPILmodel/MeasFunc/Function-Call Subsystem2 ==
  HallSpdCalc : TriggerPort  TriggerType=function-call  VariantControl=Variant
  Chart : Stateflow chart  TreatAsAtomicUnit=on
  Data Store Read3 : DataStoreRead  DataStoreName=HallPulse
  Data Store Write : DataStoreWrite  DataStoreName=HallSpd
  Data Type Conversion : DataTypeConversion  OutDataTypeStr=single
  Gain : Gain  Gain=0.1
  wires:
  Chart/1(SumOfArray) -> Gain/1
  Gain/1 -> Data Type Conversion/1
  Data Type Conversion/1 -> Data Store Write/1
  Data Store Read3/1 -> Chart/1(HallDecode)

== stateflow chart BLDCctrlBasedOnMBDPILmodel/FaultFunc/Chart ==
  state LEDoff
    (default) -> (junction 19) : {LED_OnOff = false;}
    (junction 19) -> (junction 22) : {ReadyFaultFlag = false;}
  state LEDon
    (default) -> (junction 41) : {LED_OnOff = true;}
    (junction 41) -> (junction 38) : {ReadyFaultFlag = false;}
  (default) -> LEDoff
  LEDoff -> LEDon : after(500, tick)
  LEDon -> LEDoff : after(500, tick)
  data: LED_OnOff output boolean; ReadyFaultFlag output boolean

== stateflow chart BLDCctrlBasedOnMBDPILmodel/MeasFunc/Chart ==
  (default) -> (junction 1) : {ReadSignals;}
  (junction 1) -> (junction 3) : {HallDecoder;}
  (junction 3) -> (junction 5) : {HallSpdCalc;}
  events: ReadSignals output FUNCTION_CALL_EVENT; HallDecoder output FUNCTION_CALL_EVENT; HallSpdCalc output FUNCTION_CALL_EVENT

== stateflow chart BLDCctrlBasedOnMBDPILmodel/MeasFunc/Function-Call Subsystem2/Chart ==
  (default) -> (junction 20)
  (junction 20) -> (junction 1) : [Index > 99]{Index = 0;}
  (junction 1) -> (junction 11) : {RcdArray(Index) = HallDecode;}
  (junction 11) -> (junction 14) : {Index = Index + 1;}
  (junction 14) -> (junction 17) : {SumOfArray = sum(RcdArray);}
  data: Index local uint16 =uint16(0); RcdArray local uint8 size=100; SumOfArray output double; HallDecode input

== matlab function BLDCctrlBasedOnMBDPILmodel/NomalRunFunc/Truth Table ==
  data: Hallsum input single; DutyA output single; DutyB output single; DutyC output single; DutyReq input single; DutyOffFlag output single
function [DutyA, DutyB, DutyC, DutyOffFlag] = fcn(Hallsum, DutyReq)

aVarTruthTableCondition_1 = false;
aVarTruthTableCondition_2 = false;
aVarTruthTableCondition_3 = false;
aVarTruthTableCondition_4 = false;
aVarTruthTableCondition_5 = false;
aVarTruthTableCondition_6 = false;


% Condition #1
aVarTruthTableCondition_1 = logical(Hallsum == 1);

% Condition #2
aVarTruthTableCondition_2 = logical(Hallsum == 2);

% Condition #3
aVarTruthTableCondition_3 = logical(Hallsum == 3);

% Condition #4
aVarTruthTableCondition_4 = logical(Hallsum == 4);

% Condition #5
aVarTruthTableCondition_5 = logical(Hallsum == 5);

% Condition #6
aVarTruthTableCondition_6 = logical(Hallsum == 6);

if (aVarTruthTableCondition_1 && ~aVarTruthTableCondition_2 && ~aVarTruthTableCondition_3 && ~aVarTruthTableCondition_4 && ~aVarTruthTableCondition_5 && ~aVarTruthTableCondition_6)
    aFcnTruthTableAction_1();
elseif (~aVarTruthTableCondition_1 && aVarTruthTableCondition_2 && ~aVarTruthTableCondition_3 && ~aVarTruthTableCondition_4 && ~aVarTruthTableCondition_5 && ~aVarTruthTableCondition_6)
    aFcnTruthTableAction_2();
elseif (~aVarTruthTableCondition_1 && ~aVarTruthTableCondition_2 && aVarTruthTableCondition_3 && ~aVarTruthTableCondition_4 && ~aVarTruthTableCondition_5 && ~aVarTruthTableCondition_6)
    aFcnTruthTableAction_3();
elseif (~aVarTruthTableCondition_1 && ~aVarTruthTableCondition_2 && ~aVarTruthTableCondition_3 && aVarTruthTableCondition_4 && ~aVarTruthTableCondition_5 && ~aVarTruthTableCondition_6)
    aFcnTruthTableAction_4();
elseif (~aVarTruthTableCondition_1 && ~aVarTruthTableCondition_2 && ~aVarTruthTableCondition_3 && ~aVarTruthTableCondition_4 && aVarTruthTableCondition_5 && ~aVarTruthTableCondition_6)
    aFcnTruthTableAction_5();
elseif (~aVarTruthTableCondition_1 && ~aVarTruthTableCondition_2 && ~aVarTruthTableCondition_3 && ~aVarTruthTableCondition_4 && ~aVarTruthTableCondition_5 && aVarTruthTableCondition_6)
    aFcnTruthTableAction_6();
else % Default
    aFcnTruthTableAction_7();
end

function aFcnTruthTableAction_1()

% Example action 1 called from D1 & D2 column in condition table

DutyA = DutyReq;
DutyB = 0;
DutyC = 0;
DutyOffFlag = 2;

function aFcnTruthTableAction_2()

% Example action 2 called from D3 column in condition table

DutyA = 0;
DutyB = DutyReq;
DutyC = 0;
DutyOffFlag = 3;

function aFcnTruthTableAction_3()



DutyA = 0;
DutyB = DutyReq;
DutyC = 0;
DutyOffFlag = 1;

function aFcnTruthTableAction_4()



DutyA = 0;
DutyB = 0;
DutyC = DutyReq;
DutyOffFlag = 1;

function aFcnTruthTableAction_5()



DutyA = DutyReq;
DutyB = 0;
DutyC = 0;
DutyOffFlag = 3;

function aFcnTruthTableAction_6()



DutyA = 0;
DutyB = 0;
DutyC = DutyReq;
DutyOffFlag = 2;

function aFcnTruthTableAction_7()



DutyA = 0;
DutyB = 0;
DutyC = 0;
DutyOffFlag = 0;

== stateflow chart BLDCctrlBasedOnMBDPILmodel/InitFunc/Chart ==
  (default) -> (junction 17) : {ClearVariables;}
  (junction 17) -> (junction 19) : {LED_OnOff = false;}
  (junction 19) -> (junction 22) : {InitFaultFlag = false;}
  data: LED_OnOff output boolean; InitFaultFlag output boolean
  events: ClearVariables output FUNCTION_CALL_EVENT

== stateflow chart BLDCctrlBasedOnMBDPILmodel/ReadyFunc/Chart ==
  state LEDoff
    (default) -> (junction 19) : {LED_OnOff = true;}
    (junction 19) -> (junction 22) : {ReadyFaultFlag = false;}
  state LEDon
    (default) -> (junction 41) : {LED_OnOff = false;}
    (junction 41) -> (junction 38) : {ReadyFaultFlag = false;}
  (default) -> LEDoff
  LEDoff -> LEDon : after(500, tick)
  LEDon -> LEDoff : after(500, tick)
  data: LED_OnOff output boolean; ReadyFaultFlag output boolean

== stateflow chart BLDCctrlBasedOnMBDPILmodel/Chart ==
  state Initial
    en:
    InitFunc;
    InitDone = true;
    bind:InitFunc;
  state Ready
    en:ReadyFunc;
    du:ReadyFunc;
    bind:ReadyFunc;
  state Run
    du:MeasFunc;
    state Calibration
      en:CalCnt = 0;
      du:CalCnt = CalCnt + 1;CalFunc;
      bind:CalFunc;
    state NormalRun
      en:NormalRunFunc;
      du:NormalRunFunc;
      bind:NormalRunFunc;
    (default) -> Calibration
    Calibration -> NormalRun : [CalCnt > 1000]
  state Faults
    en:FaultFunc;
    du:FaultFunc;
    bind:FaultFunc;
  (default) -> Initial : {InitDone = false;}
  Initial -> Ready [order 1] : [InitDone]
  Ready -> Run [order 1] : [MotorOnOff]
  Run -> Ready [order 1] : [~MotorOnOff]
  Ready -> Faults [order 2] : [FaultSetClear]
  Faults -> Initial : [~FaultSetClear]
  Initial -> Faults [order 2] : [FaultSetClear]
  Run -> Faults [order 2] : [FaultSetClear]
  data: CalCnt local; InitDone local boolean; MotorOnOff input boolean; FaultSetClear input boolean
  events: MeasFunc output FUNCTION_CALL_EVENT; InitFunc output FUNCTION_CALL_EVENT; ReadyFunc output FUNCTION_CALL_EVENT; CalFunc output FUNCTION_CALL_EVENT; NormalRunFunc output FUNCTION_CALL_EVENT; FaultFunc output FUNCTION_CALL_EVENT
